simulink model "cars_simulink"  (R2024b)
settings: Solver=FixedStepDiscrete  StartTime=0.0  StopTime=10.0  RelTol=1e-3
model workspace (MAT data in the model file):
  firstWarning = 1
  originalScenarioChecksum = '1F14D54FBCEF612211E37D96E1252651'
undefined symbols (not defined in the file or in its folder): driving
libraries: drivingscenarioandsensors x5, sensorinslib x1
(part 1 of 2)
settings Model: Creator=piotr  LastModifiedBy=piotr

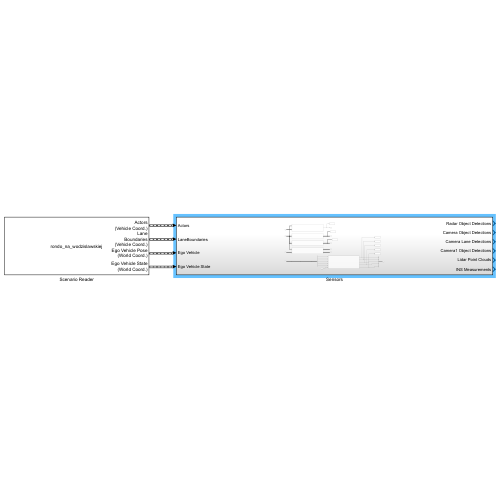
[thumbnail: Simulink's stored preview of the top-level diagram]
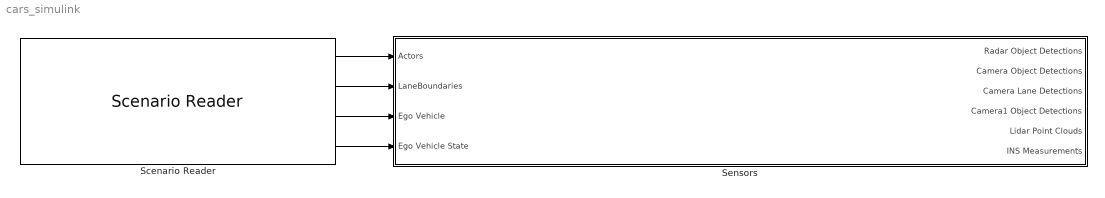
== system cars_simulink ==
  Scenario Reader : drivingscenarioandsensors/Scenario Reader  ScenarioSource=From file  ScenarioFileName=C:\Users\piotr\Desktop\Modele i Systemy Sterowania w Robotyce\MiSSwR_lab\Lab2\rondo_na_wodzislawskiej.mat  ScenarioVariableName=scenario  OutputCoordinateSystem=Vehicle coordinates  EgoVehicleSource=Scenario  EgoVehicleActorID=1  OrientVehiclesOnRoad=off  OutputEgoVehiclePose=on  OutputEgoVehicleState=on  SampleTime=0.1  LaneBoundaryOutput=Ego vehicle lane boundaries  LaneBoundaryDistance=linspace(-50, 50, 101)  LaneBoundaryLocation=Center of lane markings  BusNameSource=Auto  BusName=BusActors  BusNumActorsSource=Scenario  BusNumActors=100  BusName2Source=Auto  BusName2=BusLaneBoundaries  BusNumLaneBoundariesSource=Scenario  BusNumLaneBoundaries=10  BusName3Source=Auto  BusName3=BusEgoActor  BusName4Source=Auto  BusName4=BusEgoState  ShowCoordinateLabels=on  SimulateUsing=Interpreted execution
  Sensors : Subsystem
  wires:
  Scenario Reader/4 -> Sensors/4(Ego Vehicle State)
  Scenario Reader/3 -> Sensors/3(Ego Vehicle)
  Scenario Reader/2 -> Sensors/2(LaneBoundaries)
  Scenario Reader/1 -> Sensors/1(Actors)
